simulink model "IMUFusionSimulinkModel"  (R2020b)
settings: Solver=FixedStepDiscrete  StartTime=0.0  StopTime=1000  RelTol=1e-3
model workspace (MAT data in the model file):
  SampleRate = 100
libraries: mspfiltlib x1, mspsensorlib x1, simulink_extras x1
settings Model: Creator=The MathWorks, Inc.  LastModifiedBy=CHUNGNT28

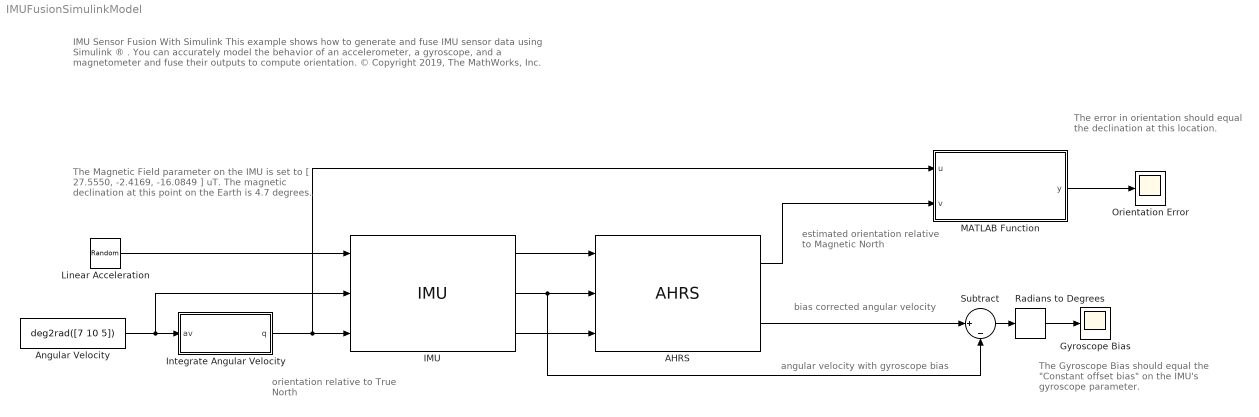
== system IMUFusionSimulinkModel ==
  note: IMU Sensor Fusion With Simulink
      | This example shows how to generate and fuse IMU sensor data using Simulink ® . You can accurately model the behavior of an accelerometer, a gyroscope, and a magnetometer and fuse their outputs to compute orientation.
      |
      | © Copyright 2019, The MathWorks, Inc.
  note: The Magnetic Field parameter on the IMU is set to
      | [ 27.5550, -2.4169, -16.0849 ] uT.
      |
      | The magnetic declination at this point
      | on the Earth is  4.7 degrees.
  note: The Gyroscope Bias should
      | equal the "Constant offset bias"
      | on the IMU's gyroscope parameter.
  note: angular velocity with gyroscope bias
  note: bias corrected angular velocity
  note: The error in orientation should
      | equal the declination at this location.
  note: estimated orientation
      | relative to Magnetic North
  note: orientation relative
      | to True North
  AHRS : mspfiltlib/AHRS  DispRefFrame=NED  DecimationFactor=1  InitialProcessNoise=ahrsfilter.defaultProcessNoise  OrientationFormat=quaternion  SimulateUsing=Code generation  AccelerometerNoise=0.0001924722  GyroscopeNoise=9.1385e-5  MagnetometerNoise=0.1  GyroscopeDriftNoise=3.0462e-13  LinearAccelerationNoise=0.0096236100000000012  MagneticDisturbanceNoise=0.5  LinearAccelerationDecayFactor=0.5  MagneticDisturbanceDecayFactor=0.5  ExpectedMagneticFieldStrength=50
      settings: SourceProductName=Sensor Fusion and Tracking Toolbox
  Angular Velocity : Constant  Value=deg2rad([7 10 5])  VectorParams1D=off  SampleTime=1/SampleRate
  Gyroscope Bias : Scope
  IMU : mspsensorlib/IMU  DispRefFrame=NED  Temperature=25  MagneticFieldNED=[ 27.5550, -2.4169, -16.0849 ]  MagneticFieldENU=[ -2.4169, 27.5550, 16.0849 ]  SeedDouble=67  SimulateUsing=Code generation  AccelParamsMeasurementRange=19.613  AccelParamsResolution=0.0023928  AccelParamsConstantBias=[0.19 0.19 0.19]  AccelParamsAxesMisalignment=[0 0 0]  AccelParamsNoiseDensity=[0.0012356 0.0012356 0.0012356]  AccelParamsBiasInstability=[0 0 0]  AccelParamsRandomWalk=[0 0 0]  AccelParamsTemperatureBias=[0 0 0]  AccelParamsTemperatureScaleFactor=[0 0 0]  GyroParamsMeasurementRange=4.3633  GyroParamsResolution=0.0011  GyroParamsConstantBias=[0.0545 0.0545 0.0545]  GyroParamsAxesMisalignment=1.5  GyroParamsAccelerationBias=[0 0 0]  GyroParamsNoiseDensity=[0.00043633 0.00043633 0.00043633]  GyroParamsBiasInstability=[0 0 0]  GyroParamsRandomWalk=[0 0 0]  GyroParamsTemperatureBias=[0 0 0]  GyroParamsTemperatureScaleFactor=[0 0 0]  MagParamsMeasurementRange=1000  MagParamsResolution=0.1  MagParamsConstantBias=0  MagParamsAxesMisalignment=[0 0 0]  MagParamsNoiseDensity=[0.0424 0.0424 0.0424]  MagParamsBiasInstability=[0 0 0]  MagParamsRandomWalk=[0 0 0]  MagParamsTemperatureBias=[0 0 0]  MagParamsTemperatureScaleFactor=[0 0 0]
      settings: SourceProductName=Sensor Fusion and Tracking Toolbox
  Integrate Angular Velocity : MATLAB Function  TreatAsAtomicUnit=on  mask{rate=SampleRate}
      mask prompts: rate "Sample Rate"
  Linear Acceleration : RandomNumber  Mean=[0 0 0]  SampleTime=1/SampleRate  VectorParams1D=off
  MATLAB Function : MATLAB Function  TreatAsAtomicUnit=on
  Orientation Error : Scope
  Radians to Degrees : simulink_extras/Transformations/Radians to Degrees
      settings: SourceProductName=Simulink Extras
  Subtract : Sum  Inputs=||+|-
  wires:
  IMU/1 -> AHRS/1
  IMU/2 -> Subtract/2, AHRS/2
  IMU/3 -> AHRS/3
  Linear Acceleration/1 -> IMU/1
  Angular Velocity/1 -> IMU/2, Integrate Angular Velocity/1(av)
  Integrate Angular Velocity/1(q) -> MATLAB Function/1(u), IMU/3
  AHRS/1 -> MATLAB Function/2(v)
  AHRS/2 -> Subtract/1
  MATLAB Function/1(y) -> Orientation Error/1
  Subtract/1 -> Radians to Degrees/1
  Radians to Degrees/1 -> Gyroscope Bias/1

== matlab function IMUFusionSimulinkModel/Integrate Angular Velocity ==
  data: av input; q output; rate parameter
function q = integrateAngVel(av, rate)
%INTEGRATEANGVEL Integrate angular velocity to a quaternion
%  Treat Angular Velocity as an incremental rotation vector.

%   Copyright 2019 The MathWorks, Inc.   

persistent orient
if isempty(orient)
    % Initial orientation is the identity quaternion.
    orient = cast(quaternion(1,0,0,0), 'like', av);
end

% Convert angular velocity to a rotation vector.
rv = quaternion(av*(1/rate), 'rotvec');
orient = rv * orient;
q = compact(orient);

== matlab function IMUFusionSimulinkModel/MATLAB Function ==
  data: u input; y output; v input
function y = orientationError(u,v)
%ORIENTATIONERROR Compute the quaternion distance in degrees

%   Copyright 2019 The MathWorks, Inc.   

y = rad2deg(dist(quaternion(u), quaternion(v)));
